simulink model "lab3_nonlinear"  (R2023a)
settings: Solver=VariableStepAuto  StartTime=0.0  StopTime=10.0  RelTol=1e-10  AbsTol=1e-10
values from neighbouring files (symbols this model uses):
  A = double(A)    [lab3.m]
  B = double(B)    [lab3.m]
  K = -K_lqr2    [lab3.m]
  Ulim = 5.875    [lab3.m]
  x0 = [0; 0; n*pi/24; 0]    [lab3.m]
settings Model: Creator=dell  LastModifiedBy=dell

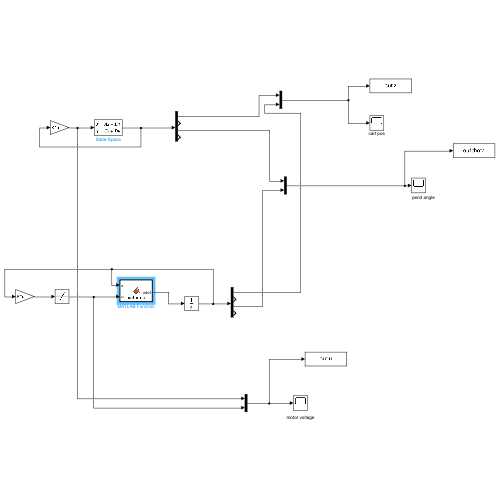
[thumbnail: Simulink's stored preview of the top-level diagram]
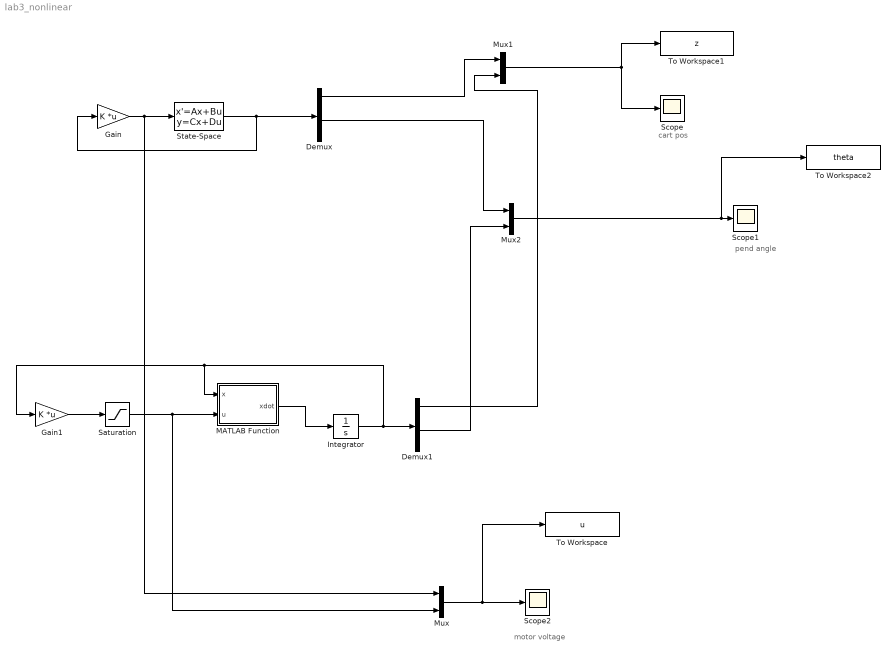
== system lab3_nonlinear ==
  note: motor voltage
  note: pend angle
  note: cart pos
  Demux : Demux
  Demux1 : Demux
  Gain : Gain  Gain=K  Multiplication=Matrix(K*u)
  Gain1 : Gain  Gain=K  Multiplication=Matrix(K*u)
  Integrator : Integrator  InitialCondition=x0
  MATLAB Function : MATLAB Function  TreatAsAtomicUnit=on
  Mux : Mux  Inputs=2
  Mux1 : Mux  Inputs=2
  Mux2 : Mux  Inputs=2
  Saturation : Saturate  UpperLimit=Ulim  LowerLimit=-Ulim
  Scope : Scope
  Scope1 : Scope
  Scope2 : Scope
  State-Space : StateSpace  A=A  B=B  C=eye(4)  D=zeros(4, 1)  InitialCondition=x0
  To Workspace : ToWorkspace  VariableName=u  SaveFormat=Timeseries  SampleTime=-1
  To Workspace1 : ToWorkspace  VariableName=z  SaveFormat=Timeseries  SampleTime=-1
  To Workspace2 : ToWorkspace  VariableName=theta  SaveFormat=Timeseries  SampleTime=-1
  wires:
  Gain/1 -> Mux/1, State-Space/1
  State-Space/1 -> Gain/1, Demux/1
  Gain1/1 -> Saturation/1
  MATLAB Function/1(xdot) -> Integrator/1
  Integrator/1 -> Gain1/1, MATLAB Function/1(x), Demux1/1
  Saturation/1 -> Mux/2, MATLAB Function/2(u)
  Mux/1 -> To Workspace/1, Scope2/1
  Demux/1 -> Mux1/1
  Mux1/1 -> To Workspace1/1, Scope/1
  Demux1/1 -> Mux1/2
  Demux1/3 -> Mux2/2
  Demux/3 -> Mux2/1
  Mux2/1 -> To Workspace2/1, Scope1/1

== matlab function lab3_nonlinear/MATLAB Function ==
  data: x input; u input; xdot output
function xdot = cartpend(x, u)
xdot = cartpend(x, u);
